simulink model "Final_model_RL"  (R2021b)
settings: Solver=FixedStepAuto  StartTime=0.0  StopTime=100  MaxStep=1e-3  RelTol=1e-3
InitFcn:
  | M = 4; D = 1.5/100; Rp = 0.05; Tg = 0.2; Ki = 1.8;
libraries: commchan3 x1
settings Model: Creator=Pooja.Aslami  LastModifiedBy=Pooja.Aslami
settings RTWCC: GenCodeOnly=on  PackageGeneratedCodeAndArtifacts=on  PackageName=simulation_code.zip
settings GRTTargetCC: CombineOutputUpdateFcns=off

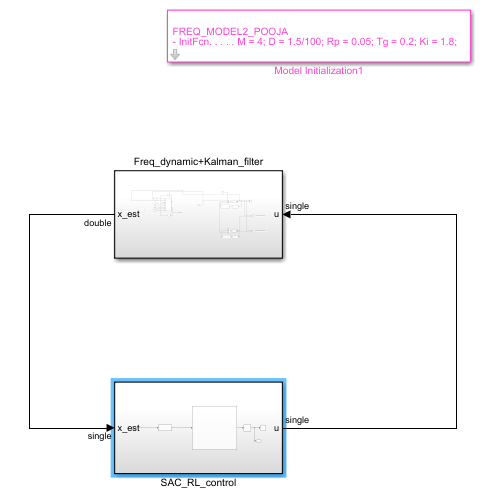
[thumbnail: Simulink's stored preview of the top-level diagram]
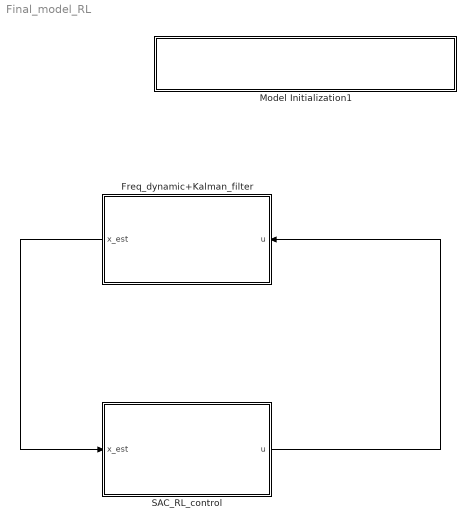
== system Final_model_RL ==
  Freq_dynamic+Kalman_filter : Subsystem
  Model Initialization1 : Subsystem  mask(Model Functions){InitFcnX=M = 4; D = 1.5/100; Rp = 0.05; Tg = 0.2; Ki = 1.8;, prel=off, posl=off, inif=on, strf=off}
      mask prompts: InitFcnX "Initialisation"; prel "Preload Function"; posl "PostLoad Function"; inif "InitFcn"; strf "StartFcn"
      mask init:
      | currentBlock = gcb;
      | root = bdroot(currentBlock);
      | 
      | if ~strcmp(get_param(root,'BlockDiagramType'),'library')
      |     if prel==1
      |         set_param(root, 'PreLoadFcn', InitFcnX);
      |     else
      |         set_param(root, 'PreLoadFcn', '');
      |     end
      |     if inif==1
      |         set_param(root, 'InitFcn', InitFcnX);
      |     else
      |         set_param(root, 'InitFcn', '');
      |     end
      |     if strf==1
      |         set_param(root, 'StartFcn', InitFcnX);
      |     else
      |         set_param(root, 'StartFcn', '');
      |     end
      |     if posl==1
      |         set_param(root, 'PostLoadFcn', InitFcnX);
      |     else
      |         set_param(root, 'PostLoadFcn', '');
      |     end
      | end
      | 
      | pos = get_param(currentBlock, 'Position');
      | width = pos(3) - pos(1); height = pos(4) - pos(2);
      | txt = [ upper(root) '\n' '- InitFcn. . . . . '  get_param(root, 'InitFcn') ];
      settings: CopyFcn=set_param(gcb,'LinkStatus','inactive')
      mask Display: text(5, height*0.5, txt, 'horizontalAlignment', 'left', 'verticalAlignment', 'middle') ;
  SAC_RL_control : Subsystem
  wires:
  Freq_dynamic+Kalman_filter/1(x_est) -> SAC_RL_control/1(x_est)
  SAC_RL_control/1(u) -> Freq_dynamic+Kalman_filter/1(u)

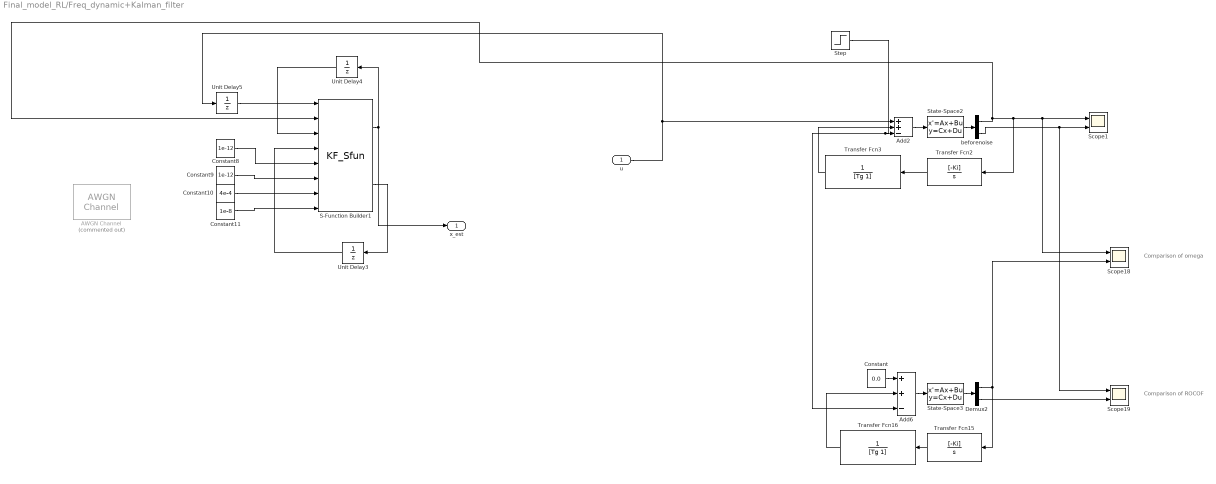
== system Final_model_RL/Freq_dynamic+Kalman_filter ==
  note: Comparison of omega
  note: Comparison of ROCOF
  u : Inport
  AWGN Channel : commchan3/AWGN Channel  Commented=on  InputProcessing=Columns as channels (frame based)  seed=65  noiseMode=Variance from mask  EbNodB=10  EsNodB=10  SNRdB=10  bitsPerSym=1  Ps=1  Tsym=1  variance=1e-8
  Add2 : Sum  Inputs=++-
  Add6 : Sum  Inputs=++-
  Constant : Constant  Value=0.0
  Constant10 : Constant  Value=4e-4
  Constant11 : Constant  Value=1e-8
  Constant8 : Constant  Value=1e-12
  Constant9 : Constant  Value=1e-12
  Demux2 : Demux  Outputs=2
  S-Function Builder1 : S-Function  InitFcn=try, set_param(gcb,'FunctionName','KF_Sfun'), end  FunctionName=KF_Sfun  SFunctionModules=KF_Sfun_wrapper EKF_Func EKF_Func_Call  SFunctionDeploymentMode=off  EnableBusSupport=off  mask(S-Function Builder){}
      mask help: Simulink:masks:SFunctionBuilder_MD
      mask init:
      | val = [[.9  0.75 0.75 1 1 .9 .9 1]',[1 1 0.75 0.75 .9 .9 1 .9]'];try , sys = get_param(gcb,'SfunBuilderFcnName');if isempty(sys), sys = get_param(gcb,'FunctionName'); end,catch, sys = get_param(gcb,'FunctionName'); end
      settings: CopyFcn=set_param(gcbh,'LinkStatus','none')  PreSaveFcn=try, set_param(gcb,'FunctionName','KF_Sfun'), end  OpenFcn=sfunctionwizard(gcbh)
      mask Display: plot(val(:,1),val(:,2)),disp(sys),port_label('input',1,'u'),port_label('input',2,'y'),port_label('input',3,'xhatp'),port_label('input',4,'Pkp'),port_label('input',5,'Q11'),port_label('input',6,'Q22'),port_label('input',7,'Q33'),port_label('input',8,'R'),port_label('output',1,'xhat'),port_label('output',2,'Phat')
  Scope1 : Scope  NumInputPorts=2
  Scope18 : Scope  NumInputPorts=2
  Scope19 : Scope  NumInputPorts=2
  State-Space2 : StateSpace  A=[0 1;-(D/(M*Tg)+1/(Rp*M*Tg)) -(D/M + 1/Tg)]  B=[0;1/(M*Tg)]  C=eye(2)  D=zeros(2,1)  InitialCondition=0
  State-Space3 : StateSpace  A=[0 1;-(D/(M*Tg)+1/(Rp*M*Tg)) -(D/M + 1/Tg)]  B=[0;1/(M*Tg)]  C=eye(2)  D=zeros(2,1)  InitialCondition=0
  Step : Step  After=0.44  SampleTime=0
  Transfer Fcn15 : TransferFcn  Numerator=[-Ki]  Denominator=[1 0]
  Transfer Fcn16 : TransferFcn  Denominator=[Tg 1]
  Transfer Fcn2 : TransferFcn  Numerator=[-Ki]  Denominator=[1 0]
  Transfer Fcn3 : TransferFcn  Denominator=[Tg 1]
  Unit Delay3 : UnitDelay  InitialCondition=1*diag([1, 1, 1])  SampleTime=0.02  HasFrameUpgradeWarning=on
  Unit Delay4 : UnitDelay  SampleTime=0.02  HasFrameUpgradeWarning=on
  Unit Delay5 : UnitDelay  SampleTime=0.02  HasFrameUpgradeWarning=on
  beforenoise : Demux  Outputs=2
  x_est : Outport
  wires:
  S-Function Builder1/2 -> Unit Delay3/1
  Unit Delay3/1 -> S-Function Builder1/4
  beforenoise/1 -> Transfer Fcn2/1, Scope18/1, Scope1/1, S-Function Builder1/2
  Step/1 -> Add6/3, Add2/3
  Constant8/1 -> S-Function Builder1/5
  Constant9/1 -> S-Function Builder1/6
  Constant10/1 -> S-Function Builder1/7
  Constant/1 -> Add6/1
  Transfer Fcn15/1 -> Transfer Fcn16/1
  Demux2/1 -> Transfer Fcn15/1, Scope18/2
  beforenoise/2 -> Scope19/1, Scope1/2
  State-Space3/1 -> Demux2/1
  Constant11/1 -> S-Function Builder1/8
  Unit Delay5/1 -> S-Function Builder1/1
  Add6/1 -> State-Space3/1
  S-Function Builder1/1 -> x_est/1, Unit Delay4/1
  Unit Delay4/1 -> S-Function Builder1/3
  State-Space2/1 -> beforenoise/1
  u/1 -> Unit Delay5/1, Add2/1
  Transfer Fcn16/1 -> Add6/2
  Transfer Fcn3/1 -> Add2/2
  Transfer Fcn2/1 -> Transfer Fcn3/1
  Add2/1 -> State-Space2/1
  Demux2/2 -> Scope19/2

== system Final_model_RL/Model Initialization1 ==

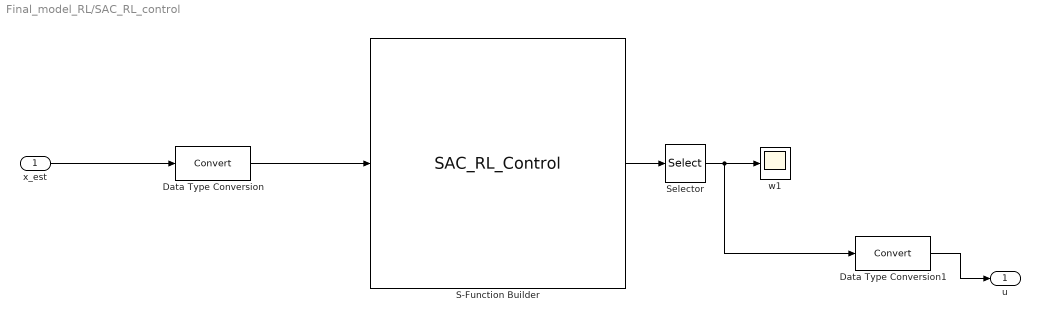
== system Final_model_RL/SAC_RL_control ==
  x_est : Inport
  Data Type Conversion : DataTypeConversion
  Data Type Conversion1 : DataTypeConversion
  S-Function Builder : S-Function  FunctionName=SAC_RL_Control  SFunctionModules=SAC_RL_Control_wrapper test_call cores layers  SFunctionDeploymentMode=off  EnableBusSupport=off  mask(S-Function Builder){}
      mask help: Simulink:masks:SFunctionBuilder_MD
      mask init: same as Final_model_RL/Freq_dynamic+Kalman_filter/S-Function Builder1
      settings: CopyFcn=set_param(gcbh,'LinkStatus','none')  OpenFcn=sfunctionwizard(gcbh)
      mask Display: plot(val(:,1),val(:,2)),disp(sys),port_label('input',1,'xhat'),port_label('output',1,'u')
  Selector : Selector  InputPortWidth=256  IndexOptions=Index vector (dialog)  Indices=[1]  OutputSizes=1
  w1 : Scope
  u : Outport
  wires:
  S-Function Builder/1 -> Selector/1
  Selector/1 -> Data Type Conversion1/1, w1/1
  x_est/1 -> Data Type Conversion/1
  Data Type Conversion/1 -> S-Function Builder/1
  Data Type Conversion1/1 -> u/1
